simulink model "validation"  (R2019a)
settings: Solver=VariableStepAuto  StartTime=0.0  StopTime=10.0  RelTol=1e-3
values from neighbouring files (symbols this model uses):
  Kp_id = 10    [nomalization.m]
  r = 60    [nomalization.m]
  r_cyc = 4000*ts    (= 200)    [nomalization.m]
undefined symbols (not defined in the file or in its folder): T_id
settings Model: Creator=xde12  LastModifiedBy=xde12

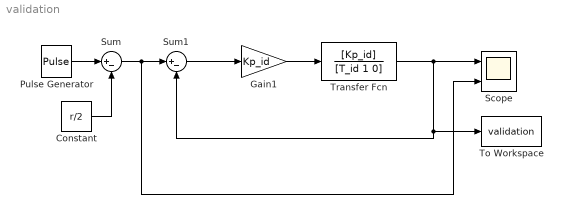
== system validation ==
  Constant : Constant  Value=r/2  SampleTime=0.01
  Gain1 : Gain  Gain=Kp_id
  Pulse Generator : DiscretePulseGenerator  PulseType=Time based  Amplitude=r  Period=r_cyc  PulseWidth=r_cyc/2  SampleTime=0.01
  Scope : Scope  NumInputPorts=2
  Sum : Sum  Inputs=|+-
  Sum1 : Sum  Inputs=|+-
  To Workspace : ToWorkspace  VariableName=validation  SampleTime=-1
      settings: Save2DSignal=2-D array (concatenate along first dimension)
  Transfer Fcn : TransferFcn  Numerator=[Kp_id]  Denominator=[T_id 1 0]
  wires:
  Constant/1 -> Sum/2
  Pulse Generator/1 -> Sum/1
  Sum1/1 -> Gain1/1
  Gain1/1 -> Transfer Fcn/1
  Transfer Fcn/1 -> To Workspace/1, Sum1/2, Scope/1
  Sum/1 -> Scope/2, Sum1/1
